simulink model "PKE_expr"  (R2014b)
settings: Solver=ode45  StartTime=0.0  StopTime=100  RelTol=1e-3
values from neighbouring files (symbols this model uses):
  B = sum(bet)    [param.m]
  bet = [2.29E-4; 8.32E-4; 7.1E-4; 8.52E-4; 1.71E-4; 1.02E-4]    [param.m]
  L = 0.00033    [param.m]
  lam = [0.0126; 0.0337; 0.139; 0.325; 1.13; 2.50]    [param.m]
  reac = B - rho    [param.m]
  t_C = 3.28    [param.m]
  t_L = 5.85    [param.m]
  y0 = [nt; Ct']    [param.m]
settings Model: Creator=VIKRAM SINGH  LastModifiedBy=VIKRAM SINGH
settings DataIOCC: LimitDataPoints=off

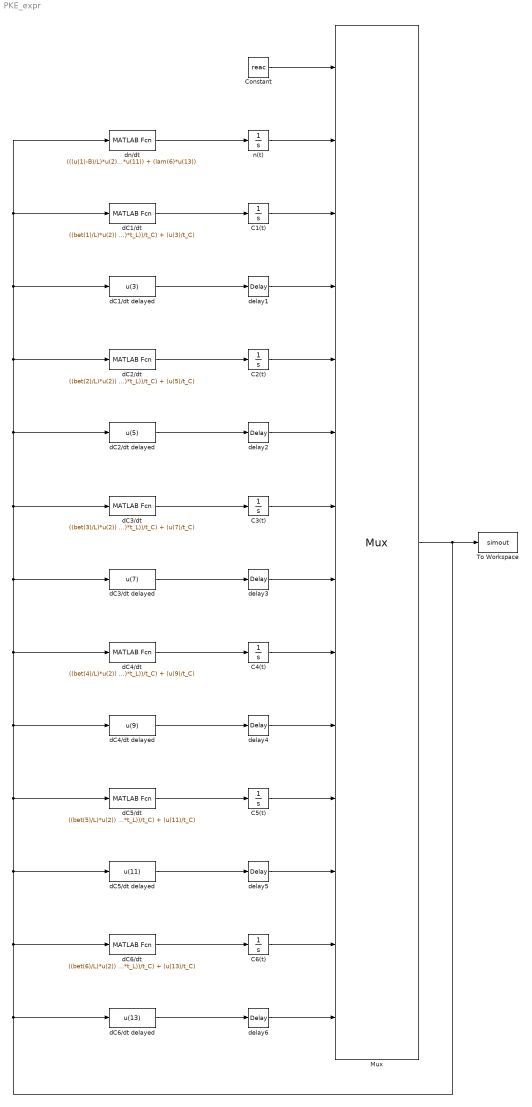
== system PKE_expr ==
  C1(t) : Integrator  InitialCondition=y0(2)
  C2(t) : Integrator  InitialCondition=y0(3)
  C3(t) : Integrator  InitialCondition=y0(4)
  C4(t) : Integrator  InitialCondition=y0(5)
  C5(t) : Integrator  InitialCondition=y0(6)
  C6(t) : Integrator  InitialCondition=y0(7)
  Constant : Constant  Value=reac
  Mux : Mux  Inputs=14
      settings: DisplayOption=signals
  To Workspace : ToWorkspace  VariableName=simout  SampleTime=-1
  dC1/dt : MATLABFcn  MATLABFcn=((bet(1)/L)*u(2)) - (lam(1)*u(3)) + ((u(4)*exp(-lam(1)*t_L))/t_C) + (u(3)/t_C)
  dC1/dt delayed : MATLABFcn  MATLABFcn=u(3)
  dC2/dt : MATLABFcn  MATLABFcn=((bet(2)/L)*u(2)) - (lam(2)*u(5)) + ((u(6)*exp(-lam(2)*t_L))/t_C) + (u(5)/t_C)
  dC2/dt delayed : MATLABFcn  MATLABFcn=u(5)
  dC3/dt : MATLABFcn  MATLABFcn=((bet(3)/L)*u(2)) - (lam(3)*u(7)) + ((u(8)*exp(-lam(3)*t_L))/t_C) + (u(7)/t_C)
  dC3/dt delayed : MATLABFcn  MATLABFcn=u(7)
  dC4/dt : MATLABFcn  MATLABFcn=((bet(4)/L)*u(2)) - (lam(4)*u(9)) + ((u(10)*exp(-lam(4)*t_L))/t_C) + (u(9)/t_C)
  dC4/dt delayed : MATLABFcn  MATLABFcn=u(9)
  dC5/dt : MATLABFcn  MATLABFcn=((bet(5)/L)*u(2)) - (lam(5)*u(11)) + ((u(12)*exp(-lam(5)*t_L))/t_C) + (u(11)/t_C)
  dC5/dt delayed : MATLABFcn  MATLABFcn=u(11)
  dC6/dt : MATLABFcn  MATLABFcn=((bet(6)/L)*u(2)) - (lam(6)*u(13)) + ((u(14)*exp(-lam(6)*t_L))/t_C) + (u(13)/t_C)
  dC6/dt delayed : MATLABFcn  MATLABFcn=u(13)
  delay1 : TransportDelay  DelayTime=t_L  InitialOutput=y0(2)
  delay2 : TransportDelay  DelayTime=t_L  InitialOutput=y0(3)
  delay3 : TransportDelay  DelayTime=t_L  InitialOutput=y0(4)
  delay4 : TransportDelay  DelayTime=t_L  InitialOutput=y0(5)
  delay5 : TransportDelay  DelayTime=t_L  InitialOutput=y0(6)
  delay6 : TransportDelay  DelayTime=t_L  InitialOutput=y0(7)
  dn/dt : MATLABFcn  MATLABFcn=(((u(1)-B)/L)*u(2)) + (lam(1)*u(3)) + (lam(2)*u(5)) + (lam(3)*u(7)) + (lam(4)*u(9)) + (lam(5)*u(11)) + (lam(6)*u(13))
  n(t) : Integrator  InitialCondition=y0(1)
  wires:
  dn/dt/1 -> n(t)/1
  dC1/dt/1 -> C1(t)/1
  Constant/1 -> Mux/1
  n(t)/1 -> Mux/2
  C1(t)/1 -> Mux/3
  dC1/dt delayed/1 -> delay1/1
  delay1/1 -> Mux/4
  dC2/dt/1 -> C2(t)/1
  C2(t)/1 -> Mux/5
  dC2/dt delayed/1 -> delay2/1
  delay2/1 -> Mux/6
  dC3/dt/1 -> C3(t)/1
  C3(t)/1 -> Mux/7
  dC3/dt delayed/1 -> delay3/1
  delay3/1 -> Mux/8
  dC4/dt/1 -> C4(t)/1
  C4(t)/1 -> Mux/9
  dC4/dt delayed/1 -> delay4/1
  delay4/1 -> Mux/10
  dC5/dt/1 -> C5(t)/1
  dC5/dt delayed/1 -> delay5/1
  C5(t)/1 -> Mux/11
  delay5/1 -> Mux/12
  dC6/dt/1 -> C6(t)/1
  dC6/dt delayed/1 -> delay6/1
  C6(t)/1 -> Mux/13
  delay6/1 -> Mux/14
  Mux/1 -> To Workspace/1, dC5/dt/1, dC4/dt delayed/1, dC4/dt/1, dC2/dt delayed/1, dC1/dt delayed/1, dn/dt/1, dC1/dt/1, dC2/dt/1, dC3/dt/1, dC3/dt delayed/1, dC5/dt delayed/1, dC6/dt/1, dC6/dt delayed/1
